simulink model "microchip_mcb_pmsm_foc_qep"  (R2021b)
settings: Solver=FixedStepDiscrete  StartTime=0.0  StopTime=8  FixedStep=Ts/2  RelTol=1e-3  EnableMultiTasking=on
InitFcn:
  | microchip_mcb_pmsm_foc_qep_data
values from neighbouring files (symbols this model uses):
  inverter = mcb_SetInverterParameters('Microchip_inverter')    [microchip_mcb_pmsm_foc_qep_data.m]
  PI_params = mcb.internal.SetControllerParameters(pmsm,inverter,PU_System,T_pwm,2*Ts,Ts_speed)    [microchip_mcb_pmsm_foc_qep_data.m]
  pmsm = mcb_SetPMSMMotorParameters('Microchip_motor')    [microchip_mcb_pmsm_foc_qep_data.m]
  PU_System = mcb_SetPUSystem(pmsm,inverter)    [microchip_mcb_pmsm_foc_qep_data.m]
  PWM_frequency = 20e3    (= 20000)    [microchip_mcb_pmsm_foc_qep_data.m]
  Ts = T_pwm    (= 5e-05)    [microchip_mcb_pmsm_foc_qep_data.m]
  Ts_motor = T_pwm/2    (= 2.5e-05)    [microchip_mcb_pmsm_foc_qep_data.m]
  Ts_simulink = T_pwm/2    (= 2.5e-05)    [microchip_mcb_pmsm_foc_qep_data.m]
  Ts_speed = 10*Ts    (= 0.0005)    [microchip_mcb_pmsm_foc_qep_data.m]
undefined symbols (not defined in the file or in its folder): A24, AD10, AD7, ADC0, LQFP144, MaxPer, ms, ns, PA0, PA1, PA10, PA11, PA12, PA13, PA18, PA9, PB0, PD18, PD19, PD24, PD25, PD26, Pin, Resol, SAME70Q21B, Unsigned, Vd_Ref_openLoop_PU
libraries: mcbcontrolslib x15, MCHP_Blockset x12, simulink x11, mcbpositiondecoderlib x4, mcbplantlib x1, autolibpmsmexterior x1
(part 1 of 4)
settings Model: Creator=Lubin Kerhuel  LastModifiedBy=Lubin Kerhuel
settings SolverCC: AlgebraicLoopSolver=TrustRegion
settings DataIOCC: SaveFormat=StructureWithTime  ReturnWorkspaceOutputs=off
settings OptimizationCC: DefaultParameterBehavior=Inlined  DefaultUnderspecifiedDataType=single  EnhancedBackFolding=on  PassReuseOutputArgsAs=Individual arguments  OptimizeBlockOrder=speed  DifferentSizesBufferReuse=on  OptimizationCustomize=off  EfficientTunableParamExpr=on
settings DebuggingCC: MultiTaskDSMMsg=none  ParameterTunabilityLossMsg=error  FcnCallInpInsideContextMsg=warning  SFExecutionAtInitializationDiag=none  SFMachineParentedDataDiag=warning  ArithmeticOperatorsInVariantConditions=warning
settings HardwareCC: ProdBitPerPointer=32  ProdBitPerSizeT=32  ProdBitPerPtrDiffT=32  ProdLargestAtomicInteger=Integer  ProdWordSize=32  ProdLongLongMode=on  ProdHWDeviceType=ARM Compatible->ARM Cortex
settings ModelReferenceCC: ModelReferenceNumInstancesAllowed=Single  PropagateSignalLabelsOutOfModel=off
settings SFSimCC: SimUseLocalCustomCode=off  MATLABDynamicMemAlloc=off  CustomCodeUndefinedFunction=UseInterfaceOnly
settings RTWCC: Description=Microchip Embedded Target Cortex M7 (real-time)  SystemTargetFile=MCHP_ARM7_stf.tlc  TemplateMakefile=MCHP_ARM7.tmf  GenerateReport=on  RTWUseLocalCustomCode=off  Toolchain=xc32 - v3.01 for Mirochip SAMx7 device  BuildConfiguration=Specify  IncludeHyperlinkInReport=on  GenerateTraceInfo=on  GenerateTraceReport=on  GenerateTraceReportSl=on  GenerateTraceReportSf=on  GenerateTraceReportEml=on
settings CodeAppCC: ForceParamTrailComments=on  IgnoreCustomStorageClasses=off  MaxIdLength=255  OperatorAnnotations=on  SimulinkDataObjDesc=on  SFDataObjDesc=on  InsertBlockDesc=on  InternalIdentifier=Classic
settings STFCustomTargetCC: MultiwordLength=256  IncludeMdlTerminateFcn=off  CombineOutputUpdateFcns=on  CombineSignalStateStructs=on  SuppressErrorStatus=on  ERTCustomFileBanners=on  SupportContinuousTime=off  RemoveResetFunc=on  MATLABClassNameForMDSCustomization=Simulink.SoftwareTarget.ERTCustomization  GRTInterface=off  UseToolchainInfoCompliant=on  SystemTargetFile=MCHP_ARM7_stf.tlc
settings ERTTargetCC: ParMdlRefBuildCompliant=off  CompOptLevelCompliant=off  ConcurrentExecutionCompliant=off  IncludeMdlTerminateFcn=off  CombineSignalStateStructs=on  SuppressErrorStatus=on  SupportNonInlinedSFcns=on  ModelStepFunctionPrototypeControlCompliant=off  CPPClassGenCompliant=off  ExtModeStaticAllocSize=2000  InlinedParameterPlacement=NonHierarchical  ERTSrcFileBannerTemplate=MCHP_dsPIC_code_template.cgt  ERTHdrFileBannerTemplate=MCHP_dsPIC_code_template.cgt  ERTDataSrcFileTemplate=MCHP_dsPIC_code_template.cgt  ERTDataHdrFileTemplate=MCHP_dsPIC_code_template.cgt  ERTCustomFileTemplate=MCHP_main.tlc

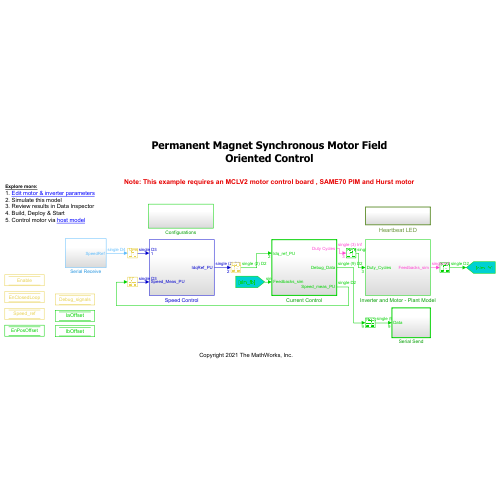
[thumbnail: Simulink's stored preview of the top-level diagram]
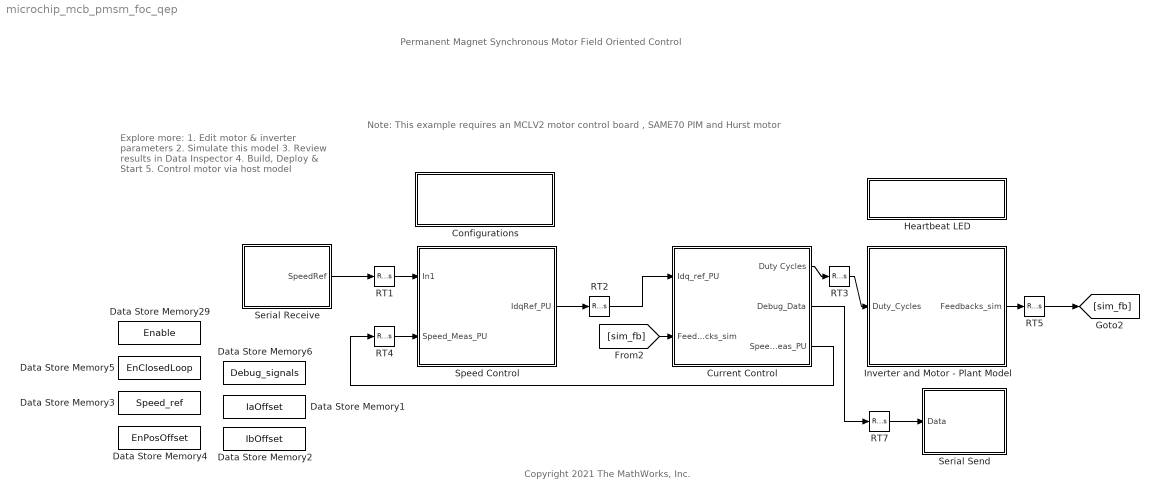
== system microchip_mcb_pmsm_foc_qep ==
  note: Permanent Magnet Synchronous Motor Field Oriented Control
  note: Copyright 2021 The MathWorks, Inc.
  note: Explore more:
      | 1. Edit motor & inverter parameters
      | 2. Simulate this model
      | 3. Review results in Data Inspector
      | 4. Build, Deploy & Start
      | 5. Control motor via host model
  note: Note: This example requires an MCLV2 motor control board , SAME70 PIM and Hurst motor
  Configurations : Subsystem
  Current Control : Subsystem  TreatAsAtomicUnit=on
  Data Store Memory1 : DataStoreMemory  DataStoreName=IaOffset  InitialValue=inverter.CtSensAOffset  ShowAdditionalParam=off
  Data Store Memory2 : DataStoreMemory  DataStoreName=IbOffset  InitialValue=inverter.CtSensBOffset  ShowAdditionalParam=off
  Data Store Memory29 : DataStoreMemory  DataStoreName=Enable  ReadBeforeWriteMsg=warning  WriteAfterWriteMsg=warning  WriteAfterReadMsg=warning  ShowAdditionalParam=off  OutDataTypeStr=boolean
  Data Store Memory3 : DataStoreMemory  DataStoreName=Speed_ref  ReadBeforeWriteMsg=warning  WriteAfterWriteMsg=warning  WriteAfterReadMsg=warning  InitialValue=0.1  ShowAdditionalParam=off  OutDataTypeStr=dataType
  Data Store Memory4 : DataStoreMemory  DataStoreName=EnPosOffset  ShowAdditionalParam=off  OutDataTypeStr=boolean
  Data Store Memory5 : DataStoreMemory  DataStoreName=EnClosedLoop  ReadBeforeWriteMsg=warning  WriteAfterWriteMsg=warning  WriteAfterReadMsg=warning  ShowAdditionalParam=off  OutDataTypeStr=boolean
  Data Store Memory6 : DataStoreMemory  DataStoreName=Debug_signals  ReadBeforeWriteMsg=warning  WriteAfterWriteMsg=warning  WriteAfterReadMsg=warning  InitialValue=1  ShowAdditionalParam=off  OutDataTypeStr=uint16
  Heartbeat LED : Subsystem  TreatAsAtomicUnit=on
  Inverter and Motor - Plant Model : Subsystem
  RT1 : RateTransition  Deterministic=off  OutPortSampleTime=Ts_speed
  RT{2..3,5,7} (4 alike) : RateTransition  Deterministic=off
  RT4 : RateTransition  Deterministic=off  OutPortSampleTime=Ts_speed
  Serial Receive : Subsystem
  Serial Send : Subsystem  TreatAsAtomicUnit=on  SystemSampleTime=Ts
  Speed Control : Subsystem  SystemSampleTime=Ts_speed
  wires:
  Current Control/3(Speed_meas_PU) -> RT4/1
  Current Control/2(Debug_Data) -> RT7/1
  RT3/1 -> Inverter and Motor - Plant Model/1(Duty_Cycles)
  RT7/1 -> Serial Send/1(Data)
  RT1/1 -> Speed Control/1(In1)
  Serial Receive/1(SpeedRef) -> RT1/1
  RT2/1 -> Current Control/1(Idq_ref_PU)
  RT4/1 -> Speed Control/2(Speed_Meas_PU)
  Current Control/1(Duty Cycles) -> RT3/1
  Inverter and Motor - Plant Model/1(Feedbacks_sim) -> RT5/1
  [sim_fb] -> Current Control/2(Feedbacks_sim)
  RT5/1 -> [sim_fb]
  Speed Control/1(IdqRef_PU) -> RT2/1
